simulink model "model_harmonic"  (Simulink 7.0)
settings: Solver=ode45  StartTime=0.0  StopTime=10.0  MaxStep=0.1  RelTol=1e-3
settings Model: Creator=peter  LastModifiedBy=peter  ExtModeAutoUpdateStatusClock=off

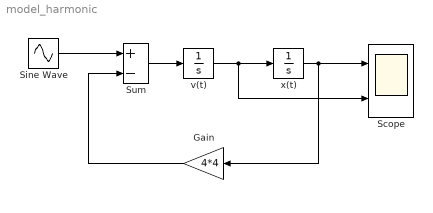
== system model_harmonic ==
  Gain : Gain  Orientation=left  Gain=4*4  ParameterDataType=sfix(16)  ParameterScaling=2^0  OutDataType=sfix(16)  OutScaling=2^0
  Scope : Scope  NumInputPorts=2
      settings: TimeRange=10  YMin=-1.1~-1.1  YMax=1.1~1.1
  Sine Wave : Sin  Frequency=3  SampleTime=0
  Sum : Sum  Inputs=+-  OutDataType=sfix(16)  OutScaling=2^0
  v(t) : Integrator
  x(t) : Integrator
  wires:
  v(t)/1 -> x(t)/1, Scope/2
  x(t)/1 -> Gain/1, Scope/1
  Sum/1 -> v(t)/1
  Gain/1 -> Sum/2
  Sine Wave/1 -> Sum/1
